simulink model "poledelay"  (R2020a)
settings: Solver=FixedStepDiscrete  StartTime=0.0  StopTime=16  FixedStep=0.6764  RelTol=1e-3
undefined symbols (not defined in the file): C, gamma, Kf, Kff, phi
settings Model: Creator=macharold  LastModifiedBy=jose
settings DataIOCC: ReturnWorkspaceOutputs=off
settings DebuggingCC: ArithmeticOperatorsInVariantConditions=warning
settings SFSimCC: SimUseLocalCustomCode=off  CustomCodeUndefinedFunction=UseInterfaceOnly
settings RTWCC: RTWUseLocalCustomCode=off

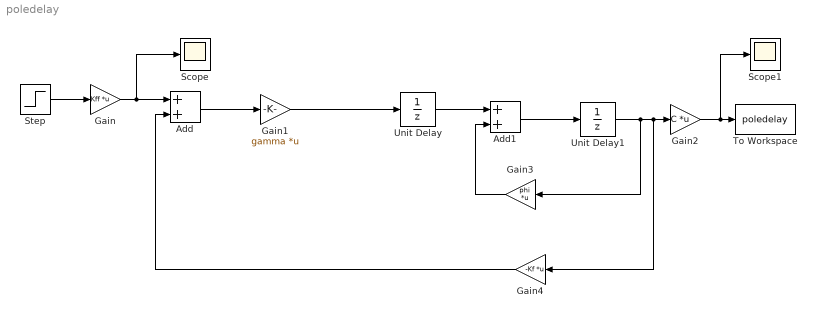
== system poledelay ==
  Add : Sum
  Add1 : Sum
  Gain : Gain  Gain=Kff  Multiplication=Matrix(K*u)
  Gain1 : Gain  Gain=gamma  Multiplication=Matrix(K*u)
  Gain2 : Gain  Gain=C  Multiplication=Matrix(K*u)
  Gain3 : Gain  Gain=phi  Multiplication=Matrix(K*u)
  Gain4 : Gain  Gain=-Kf  Multiplication=Matrix(K*u)
  Scope : Scope
  Scope1 : Scope
  Step : Step  Before=1  SampleTime=0
  To Workspace : ToWorkspace  VariableName=poledelay  SaveFormat=Timeseries  SampleTime=-1
  Unit Delay : UnitDelay  SampleTime=-1  HasFrameUpgradeWarning=on
  Unit Delay1 : UnitDelay  SampleTime=-1  HasFrameUpgradeWarning=on
  wires:
  Gain/1 -> Scope/1, Add/1
  Add/1 -> Gain1/1
  Gain1/1 -> Unit Delay/1
  Unit Delay/1 -> Add1/1
  Add1/1 -> Unit Delay1/1
  Unit Delay1/1 -> Gain3/1, Gain4/1, Gain2/1
  Gain2/1 -> Scope1/1, To Workspace/1
  Gain3/1 -> Add1/2
  Gain4/1 -> Add/2
  Step/1 -> Gain/1
